simulink model "F16_actlib"  (Simulink 6.0)
settings: Solver=ode45  StartTime=0.0  StopTime=10.0  RelTol=1e-3
values from neighbouring files (symbols this model uses):
  init_dlef = uu(5)    [runF16model.m]
  init_u = uu(1:4)    [runF16model.m]
settings Model: Creator=larssonneveldt  LastModifiedBy=larssonneveldt
settings OptimizationCC: ExpressionDepthLimit=2147483647  SimCompilerOptimization=Off
settings DebuggingCC: SaveWithParameterizedLinksMsg=none  MultiTaskDSMMsg=warning  MultiTaskCondExecSysMsg=none  FcnCallInpInsideContextMsg=Use local settings  StateNameClashWarn=warning  StrictBusMsg=None
settings HardwareCC: TargetHWDeviceType=32-bit Generic
settings RTWCC: IncludeERTFirstTime=on  RTWCompilerOptimization=Off
settings CodeAppCC: CustomSymbolStrType=$N$R$M

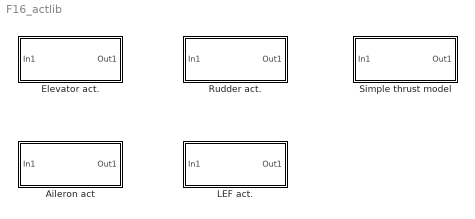
== system F16_actlib ==
  Aileron act : Subsystem
      mask Display:
      | port_label('output', 1, 'da')
      | port_label('input', 1, 'da_ref')
  Elevator act. : Subsystem
      mask Display:
      | port_label('output', 1, 'de')
      | port_label('input', 1, 'de_ref')
  LEF act. : Subsystem
      mask Display:
      | port_label('output', 1, 'dlef')
      | port_label('input', 1, 'dlef_ref')
  Rudder act. : Subsystem
      mask Display:
      | port_label('output', 1, 'dr')
      | port_label('input', 1, 'dr_ref')
  Simple thrust model : Subsystem
      mask Display:
      | port_label('output', 1, 'T')
      | port_label('input', 1, 'T_ref')

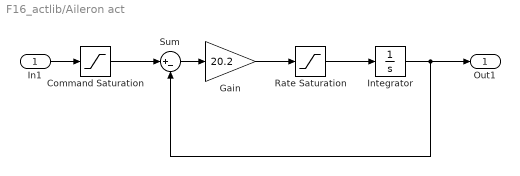
== system F16_actlib/Aileron act ==
  In1 : Inport  OutDataType=sfix(16)  OutScaling=2^0
  Command Saturation : Saturate  UpperLimit=21.5*pi/180  LowerLimit=-21.5*pi/180
  Gain : Gain  Gain=20.2  ParameterDataType=sfix(16)  ParameterScaling=2^0  OutDataType=sfix(16)  OutScaling=2^0  SaturateOnIntegerOverflow=on
  "Integrator " : Integrator  InitialCondition=init_u(3)  UpperSaturationLimit=21.5  LowerSaturationLimit=-21.5
  Rate Saturation : Saturate  UpperLimit=80*pi/180  LowerLimit=-80*pi/180
  Sum : Sum  Inputs=|+-  OutDataType=sfix(16)  OutScaling=2^0  SaturateOnIntegerOverflow=on  InputSameDT=on
  Out1 : Outport  OutDataType=sfix(16)  OutScaling=2^0
  wires:
  In1/1 -> Command Saturation/1
  Command Saturation/1 -> Sum/1
  Sum/1 -> Gain/1
  Gain/1 -> Rate Saturation/1
  Rate Saturation/1 -> "Integrator "/1
  "Integrator "/1 -> Out1/1, Sum/2

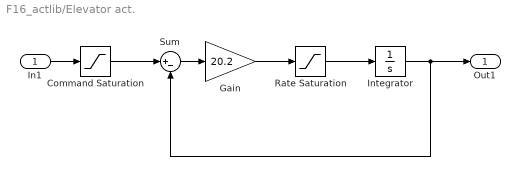
== system F16_actlib/Elevator act. ==
  In1 : Inport  OutDataType=sfix(16)  OutScaling=2^0
  Command Saturation : Saturate  UpperLimit=25*pi/180  LowerLimit=-25*pi/180
  Gain : Gain  Gain=20.2  ParameterDataType=sfix(16)  ParameterScaling=2^0  OutDataType=sfix(16)  OutScaling=2^0  SaturateOnIntegerOverflow=on
  "Integrator " : Integrator  InitialCondition=init_u(2)  UpperSaturationLimit=25  LowerSaturationLimit=-25
  Rate Saturation : Saturate  UpperLimit=60*pi/180  LowerLimit=-60*pi/180
  Sum : Sum  Inputs=|+-  OutDataType=sfix(16)  OutScaling=2^0  SaturateOnIntegerOverflow=on  InputSameDT=on
  Out1 : Outport  OutDataType=sfix(16)  OutScaling=2^0
  wires:
  In1/1 -> Command Saturation/1
  Command Saturation/1 -> Sum/1
  Sum/1 -> Gain/1
  Gain/1 -> Rate Saturation/1
  Rate Saturation/1 -> "Integrator "/1
  "Integrator "/1 -> Out1/1, Sum/2

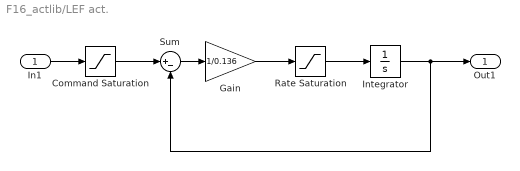
== system F16_actlib/LEF act. ==
  In1 : Inport  OutDataType=sfix(16)  OutScaling=2^0
  Command Saturation : Saturate  UpperLimit=25  LowerLimit=0
  Gain : Gain  Gain=1/0.136  ParameterDataType=sfix(16)  ParameterScaling=2^0  OutDataType=sfix(16)  OutScaling=2^0  SaturateOnIntegerOverflow=on
  "Integrator " : Integrator  InitialCondition=init_dlef  UpperSaturationLimit=25  LowerSaturationLimit=-25
  Rate Saturation : Saturate  UpperLimit=25  LowerLimit=-25
  Sum : Sum  Inputs=|+-  OutDataType=sfix(16)  OutScaling=2^0  SaturateOnIntegerOverflow=on  InputSameDT=on
  Out1 : Outport  OutDataType=sfix(16)  OutScaling=2^0
  wires:
  "Integrator "/1 -> Sum/2, Out1/1
  Rate Saturation/1 -> "Integrator "/1
  Gain/1 -> Rate Saturation/1
  Sum/1 -> Gain/1
  Command Saturation/1 -> Sum/1
  In1/1 -> Command Saturation/1

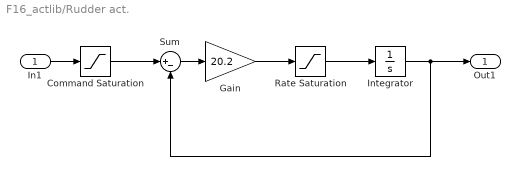
== system F16_actlib/Rudder act. ==
  In1 : Inport  OutDataType=sfix(16)  OutScaling=2^0
  Command Saturation : Saturate  UpperLimit=30*pi/180  LowerLimit=-30*pi/180
  Gain : Gain  Gain=20.2  ParameterDataType=sfix(16)  ParameterScaling=2^0  OutDataType=sfix(16)  OutScaling=2^0  SaturateOnIntegerOverflow=on
  "Integrator " : Integrator  InitialCondition=init_u(4)  UpperSaturationLimit=25  LowerSaturationLimit=-25
  Rate Saturation : Saturate  UpperLimit=120*pi/180  LowerLimit=-120*pi/180
  Sum : Sum  Inputs=|+-  OutDataType=sfix(16)  OutScaling=2^0  SaturateOnIntegerOverflow=on  InputSameDT=on
  Out1 : Outport  OutDataType=sfix(16)  OutScaling=2^0
  wires:
  "Integrator "/1 -> Sum/2, Out1/1
  Rate Saturation/1 -> "Integrator "/1
  Gain/1 -> Rate Saturation/1
  Sum/1 -> Gain/1
  Command Saturation/1 -> Sum/1
  In1/1 -> Command Saturation/1

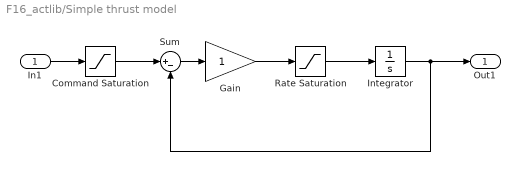
== system F16_actlib/Simple thrust model ==
  In1 : Inport  OutDataType=sfix(16)  OutScaling=2^0
  Command Saturation : Saturate  UpperLimit=85000  LowerLimit=4500
  Gain : Gain  ParameterDataType=sfix(16)  ParameterScaling=2^0  OutDataType=sfix(16)  OutScaling=2^0  SaturateOnIntegerOverflow=on
  "Integrator " : Integrator  InitialCondition=init_u(1)  UpperSaturationLimit=45000  LowerSaturationLimit=-45000
  Rate Saturation : Saturate  UpperLimit=45000  LowerLimit=-45000
  Sum : Sum  Inputs=|+-  OutDataType=sfix(16)  OutScaling=2^0  SaturateOnIntegerOverflow=on  InputSameDT=on
  Out1 : Outport  OutDataType=sfix(16)  OutScaling=2^0
  wires:
  In1/1 -> Command Saturation/1
  Command Saturation/1 -> Sum/1
  Sum/1 -> Gain/1
  Gain/1 -> Rate Saturation/1
  Rate Saturation/1 -> "Integrator "/1
  "Integrator "/1 -> Out1/1, Sum/2
